simulink model "mux_3channels"  (Simulink 6.6)
settings: Solver=ode45  StartTime=0.0  StopTime=35  RelTol=1e-3
undefined symbols (not defined in the file): A, B, D, PCIN, X, Z
libraries: xbsIndex_r4 x50
settings Model: Creator=lcrockett  LastModifiedBy=lcrockett

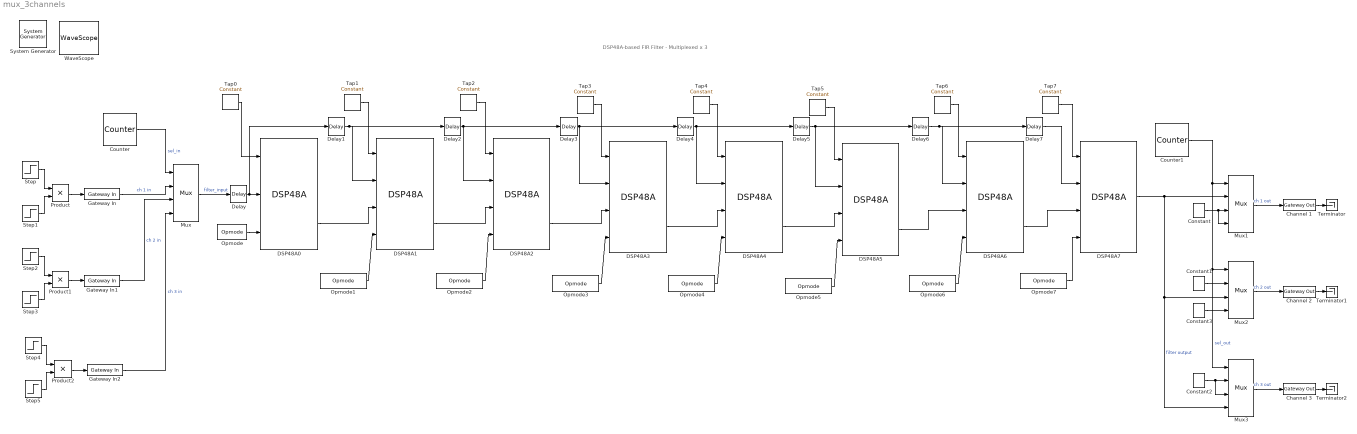
== system mux_3channels ==
  note: DSP48A-based FIR Filter - Multiplexed x 3
  " System Generator" : xbsIndex_r4/ System Generator  Tag=genX  SystemSampleTime=-1  xilinxfamily=spartan3adsp  part=xc3sd1800a  speed=-5  package=cs484  synthesis_tool=XST  clock_wrapper=Clock Enables  directory=./mux3  testbench=off  simulink_period=1  sysclk_period=5  dcm_input_clock_period=100  incr_netlist=off  trim_vbits=Everywhere in SubSystem  dbl_ovrd=According to Block Masks  core_generation=According to Block Masks  run_coregen=off  deprecated_control=off  eval_field=0  block_type=sysgen
      settings: block_version=9.2.01
  Channel 1 : xbsIndex_r4/Gateway Out  hdl_port=on  timing_constraint=None  locs_specified=off  LOCs={}  block_type=gatewayout
      settings: infoedit="Gateway out block.  Converts Xilinx fixed point inputs into ouputs of type Simulink integer, double, or fixed point.<P><P>Hardware notes:  In hardware these blocks become top level output ports or are discarded, depending on how they are configured."  block_version=9.2.01
  Channel 2 : xbsIndex_r4/Gateway Out  hdl_port=on  timing_constraint=None  locs_specified=off  LOCs={}  block_type=gatewayout
      settings: infoedit="Gateway out block.  Converts Xilinx fixed point inputs into ouputs of type Simulink integer, double, or fixed point.<P><P>Hardware notes:  In hardware these blocks become top level output ports or are discarded, depending on how they are configured."  block_version=9.2.01
  Channel 3 : xbsIndex_r4/Gateway Out  hdl_port=on  timing_constraint=None  locs_specified=off  LOCs={}  block_type=gatewayout
      settings: infoedit="Gateway out block.  Converts Xilinx fixed point inputs into ouputs of type Simulink integer, double, or fixed point.<P><P>Hardware notes:  In hardware these blocks become top level output ports or are discarded, depending on how they are configured."  block_version=9.2.01
  Constant{,1..3} (4 alike) : xbsIndex_r4/Constant  arith_type=Signed (2's comp)  const=0  n_bits=18  bin_pt=0  explicit_period=off  period=1  equ=P=C  opselect=C  inp2=PCIN>>17  opr=+  inp1=P  carry=CIN  dbl_ovrd=off  block_type=constant
      settings: block_version=9.2.01
  Counter : xbsIndex_r4/Counter  cnt_type=Count Limited  cnt_to=2  operation=Up  start_count=0  cnt_by_val=1  arith_type=Unsigned  n_bits=2  bin_pt=0  load_pin=off  rst=off  en=off  explicit_period=on  period=1  dbl_ovrd=off  use_behavioral_HDL=off  use_rpm=off  block_type=counter
      settings: block_version=9.2.01
  Counter1 : xbsIndex_r4/Counter  cnt_type=Count Limited  cnt_to=2  operation=Up  start_count=0  cnt_by_val=1  arith_type=Unsigned  n_bits=2  bin_pt=0  load_pin=off  rst=off  en=off  explicit_period=on  period=1  dbl_ovrd=off  use_behavioral_HDL=off  use_rpm=off  block_type=counter
      settings: block_version=9.2.01
  DSP48A0 : xbsIndex_r4/DSP48A  use_op=on  use_creg=off  use_d=off  use_pcin=off  use_pcout=on  use_bcout=off  use_carryin=off  use_carryout=off  rst_all=off  en_all=off  carryin_type=Direct from carry in port  use_a0reg=on  use_a1reg=off  use_b0reg=on  use_b1reg=off  pipeline_c=on  pipeline_d=off  pipeline_mult=on  pipeline_p=off  pipeline_opmode=on  pipeline_carryin=on  rst_a=off  rst_b=off  rst_c=off  rst_d=off  rst_mult=off  rst_p=off  rst_opmode=off  rst_carry_in=off  en_a=off  en_b=off  en_c=off  en_d=off  en_mult=off  en_p=off  en_opmode=off  en_carry_in=off  dbl_ovrd=off  use_synth_model=off  device=3  block_type=dsp48a
      settings: block_version=9.2.01
  DSP48A{1..6} (6 alike) : xbsIndex_r4/DSP48A  use_op=on  use_creg=off  use_d=off  use_pcin=on  use_pcout=on  use_bcout=off  use_carryin=off  use_carryout=off  rst_all=off  en_all=off  carryin_type=Direct from carry in port  use_a0reg=on  use_a1reg=off  use_b0reg=on  use_b1reg=off  pipeline_c=on  pipeline_d=off  pipeline_mult=on  pipeline_p=off  pipeline_opmode=on  pipeline_carryin=on  rst_a=off  rst_b=off  rst_c=off  rst_d=off  rst_mult=off  rst_p=off  rst_opmode=off  rst_carry_in=off  en_a=off  en_b=off  en_c=off  en_d=off  en_mult=off  en_p=off  en_opmode=off  en_carry_in=off  dbl_ovrd=off  use_synth_model=off  device=3  block_type=dsp48a
      settings: block_version=9.2.01
  DSP48A7 : xbsIndex_r4/DSP48A  use_op=on  use_creg=off  use_d=off  use_pcin=on  use_pcout=off  use_bcout=off  use_carryin=off  use_carryout=off  rst_all=off  en_all=off  carryin_type=Direct from carry in port  use_a0reg=on  use_a1reg=off  use_b0reg=on  use_b1reg=off  pipeline_c=on  pipeline_d=off  pipeline_mult=on  pipeline_p=off  pipeline_opmode=on  pipeline_carryin=on  rst_a=off  rst_b=off  rst_c=off  rst_d=off  rst_mult=off  rst_p=off  rst_opmode=off  rst_carry_in=off  en_a=off  en_b=off  en_c=off  en_d=off  en_mult=off  en_p=off  en_opmode=off  en_carry_in=off  dbl_ovrd=off  use_synth_model=off  device=3  block_type=dsp48a
      settings: block_version=9.2.01
  Delay : xbsIndex_r4/Delay  en=off  latency=1  dbl_ovrd=off  reg_retiming=off  block_type=delay
      settings: block_version=9.2.01
  Delay{1..7} (7 alike) : xbsIndex_r4/Delay  en=off  latency=3  dbl_ovrd=off  reg_retiming=off  block_type=delay
      settings: block_version=9.2.01
  Gateway In : xbsIndex_r4/Gateway In  arith_type="Signed  (2's comp)"  n_bits=18  bin_pt=0  quantization="Round  (unbiased: +/- Inf)"  overflow=Saturate  period=1  dbl_ovrd=off  timing_constraint=None  locs_specified=off  LOCs={}  block_type=gatewayin
      settings: infoedit="Gateway in block.  Converts inputs of type Simulink integer, double and fixed point to  Xilinx fixed point type.<P><P>Hardware notes:  In hardware these blocks become top level input ports."  block_version=9.2.01
  Gateway In1 : xbsIndex_r4/Gateway In  arith_type="Signed  (2's comp)"  n_bits=18  bin_pt=0  quantization="Round  (unbiased: +/- Inf)"  overflow=Saturate  period=1  dbl_ovrd=off  timing_constraint=None  locs_specified=off  LOCs={}  block_type=gatewayin
      settings: infoedit="Gateway in block.  Converts inputs of type Simulink integer, double and fixed point to  Xilinx fixed point type.<P><P>Hardware notes:  In hardware these blocks become top level input ports."  block_version=9.2.01
  Gateway In2 : xbsIndex_r4/Gateway In  arith_type="Signed  (2's comp)"  n_bits=18  bin_pt=0  quantization="Round  (unbiased: +/- Inf)"  overflow=Saturate  period=1  dbl_ovrd=off  timing_constraint=None  locs_specified=off  LOCs={}  block_type=gatewayin
      settings: infoedit="Gateway in block.  Converts inputs of type Simulink integer, double and fixed point to  Xilinx fixed point type.<P><P>Hardware notes:  In hardware these blocks become top level input ports."  block_version=9.2.01
  Mux{,1..3} (4 alike) : xbsIndex_r4/Mux  inputs=3  en=off  latency=0  precision=Full  arith_type=Unsigned  n_bits=16  bin_pt=14  quantization=Truncate  overflow=Wrap  dbl_ovrd=off  block_type=mux
      settings: block_version=9.2.01
  Opmode : xbsIndex_r4/Opmode  device=DSP48A  equ=P=(A*B)  operation=A * B  logicinstr=X + Z  z_mux=C  operand=+  xy_mux=P  x_mux=A*(D+B)  carry=0  dbl_ovrd=off  block_type=opmode
      settings: block_version=9.2.01
  Opmode{1..7} (7 alike) : xbsIndex_r4/Opmode  device=DSP48A  equ=P=PCIN+(A*B)  operation=PCIN + A*B  logicinstr=X + Z  z_mux=P  operand=+  xy_mux=P  x_mux=A*(D+B)  carry=0  dbl_ovrd=off  block_type=opmode
      settings: block_version=9.2.01
  Product : Product  RndMeth=Zero
  Product1 : Product  RndMeth=Zero
  Product2 : Product  RndMeth=Zero
  Step : Step  Time=3  SampleTime=1
  Step1 : Step  Time=4  Before=1  After=0  SampleTime=1
  Step2 : Step  Time=4  SampleTime=1
  Step3 : Step  Time=5  Before=-2  After=0  SampleTime=1
  Step4 : Step  Time=5  SampleTime=1
  Step5 : Step  Time=6  Before=-1  After=0  SampleTime=1
  Tap0 : xbsIndex_r4/Constant  arith_type=Signed (2's comp)  const=14  n_bits=18  bin_pt=0  explicit_period=off  period=1  equ=P=C  opselect=C  inp2=PCIN>>17  opr=+  inp1=P  carry=CIN  dbl_ovrd=off  block_type=constant
      settings: block_version=9.2.01
  Tap1 : xbsIndex_r4/Constant  arith_type=Signed (2's comp)  const=64  n_bits=18  bin_pt=0  explicit_period=off  period=1  equ=P=C  opselect=C  inp2=PCIN>>17  opr=+  inp1=P  carry=CIN  dbl_ovrd=off  block_type=constant
      settings: block_version=9.2.01
  Tap2 : xbsIndex_r4/Constant  arith_type=Signed (2's comp)  const=-30  n_bits=18  bin_pt=0  explicit_period=off  period=1  equ=P=C  opselect=C  inp2=PCIN>>17  opr=+  inp1=P  carry=CIN  dbl_ovrd=off  block_type=constant
      settings: block_version=9.2.01
  Tap3 : xbsIndex_r4/Constant  arith_type=Signed (2's comp)  const=153  n_bits=18  bin_pt=0  explicit_period=off  period=1  equ=P=C  opselect=C  inp2=PCIN>>17  opr=+  inp1=P  carry=CIN  dbl_ovrd=off  block_type=constant
      settings: block_version=9.2.01
  Tap4 : xbsIndex_r4/Constant  arith_type=Signed (2's comp)  const=-99  n_bits=18  bin_pt=0  explicit_period=off  period=1  equ=P=C  opselect=C  inp2=PCIN>>17  opr=+  inp1=P  carry=CIN  dbl_ovrd=off  block_type=constant
      settings: block_version=9.2.01
  Tap5 : xbsIndex_r4/Constant  arith_type=Signed (2's comp)  const=1  n_bits=18  bin_pt=0  explicit_period=off  period=1  equ=P=C  opselect=C  inp2=PCIN>>17  opr=+  inp1=P  carry=CIN  dbl_ovrd=off  block_type=constant
      settings: block_version=9.2.01
  Tap6 : xbsIndex_r4/Constant  arith_type=Signed (2's comp)  const=-17  n_bits=18  bin_pt=0  explicit_period=off  period=1  equ=P=C  opselect=C  inp2=PCIN>>17  opr=+  inp1=P  carry=CIN  dbl_ovrd=off  block_type=constant
      settings: block_version=9.2.01
  Tap7 : xbsIndex_r4/Constant  arith_type=Signed (2's comp)  const=-25  n_bits=18  bin_pt=0  explicit_period=off  period=1  equ=P=C  opselect=C  inp2=PCIN>>17  opr=+  inp1=P  carry=CIN  dbl_ovrd=off  block_type=constant
      settings: block_version=9.2.01
  Terminator : Terminator
  Terminator1 : Terminator
  Terminator2 : Terminator
  WaveScope : xbsIndex_r4/WaveScope  block_type=wavescope
      settings: block_version=9.2.01
  wires:
  Opmode/1 -> DSP48A0/3
  Opmode1/1 -> DSP48A1/4
  DSP48A0/2 -> DSP48A1/3
  Tap1/1 -> DSP48A1/1
  Tap0/1 -> DSP48A0/1
  Product/1 -> Gateway In/1
  Step/1 -> Product/1
  Step1/1 -> Product/2
  Channel 1/1 -> Terminator/1
  Opmode2/1 -> DSP48A2/4
  DSP48A1/2 -> DSP48A2/3
  Tap2/1 -> DSP48A2/1
  Opmode3/1 -> DSP48A3/4
  DSP48A2/2 -> DSP48A3/3
  Tap3/1 -> DSP48A3/1
  Opmode4/1 -> DSP48A4/4
  DSP48A3/2 -> DSP48A4/3
  Tap4/1 -> DSP48A4/1
  Opmode5/1 -> DSP48A5/4
  DSP48A4/2 -> DSP48A5/3
  Tap5/1 -> DSP48A5/1
  Opmode6/1 -> DSP48A6/4
  Tap6/1 -> DSP48A6/1
  DSP48A5/2 -> DSP48A6/3
  Opmode7/1 -> DSP48A7/4
  DSP48A6/2 -> DSP48A7/3
  Tap7/1 -> DSP48A7/1
  Delay/1 -> DSP48A0/2, Delay1/1
  Delay1/1 -> DSP48A1/2, Delay2/1
  Delay2/1 -> DSP48A2/2, Delay3/1
  Delay3/1 -> DSP48A3/2, Delay4/1
  Delay4/1 -> DSP48A4/2, Delay5/1
  Delay5/1 -> DSP48A5/2, Delay6/1
  Delay6/1 -> DSP48A6/2, Delay7/1
  Delay7/1 -> DSP48A7/2
  Mux/1 -> Delay/1  "filter_input"
  Product1/1 -> Gateway In1/1
  Step2/1 -> Product1/1
  Step3/1 -> Product1/2
  Counter/1 -> Mux/1  "sel_in"
  Gateway In/1 -> Mux/2  "ch 1 in"
  Gateway In1/1 -> Mux/3  "ch 2 in"
  Counter1/1 -> Mux1/1, Mux2/1, Mux3/1  "sel_out"
  Mux1/1 -> Channel 1/1  "ch 1 out"
  DSP48A7/1 -> Mux1/2, Mux2/3, Mux3/4  "filter output"
  Constant/1 -> Mux1/3, Mux1/4
  Channel 2/1 -> Terminator1/1
  Mux2/1 -> Channel 2/1  "ch 2 out"
  Constant1/1 -> Mux2/2
  Product2/1 -> Gateway In2/1
  Step4/1 -> Product2/1
  Step5/1 -> Product2/2
  Gateway In2/1 -> Mux/4  "ch 3 in"
  Channel 3/1 -> Terminator2/1
  Mux3/1 -> Channel 3/1  "ch 3 out"
  Constant2/1 -> Mux3/2, Mux3/3
  Constant3/1 -> Mux2/4
